simulink model "RI_PMDC_PI"  (R2013b)
settings: Solver=ode45  StartTime=0.0  StopTime=10.0  RelTol=1e-3
libraries: RI_MK x3, simulink x1
settings Model: Creator=Szalay  LastModifiedBy=Szalay

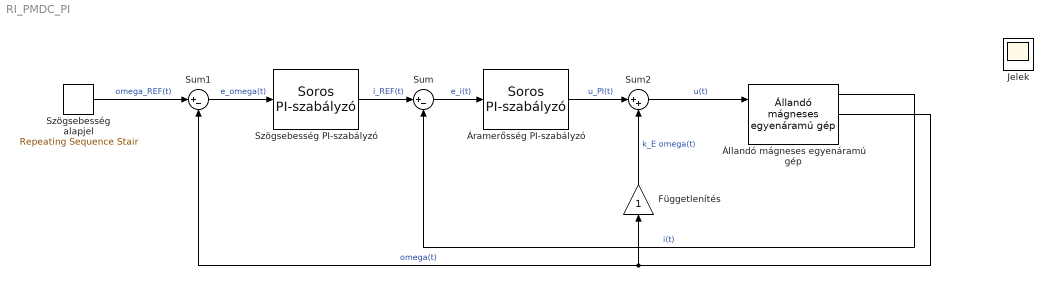
== system RI_PMDC_PI ==
  Függetlenítés : Gain
  Jelek : Scope
  Sum : Sum  Inputs=|+-
  Sum1 : Sum  Inputs=|+-
  Sum2 : Sum  Inputs=|++
  Szögsebesség PI-szabályzó : RI_MK/Soros PI-szabályzó  K_PI=1  T_I=1
  Szögsebesség alapjel : simulink/Sources/Repeating Sequence Stair  OutValues=[3 1 4 2 1].'  tsamp=-1  OutMin=[]  OutMax=[]  OutDataTypeStr=double  OutputDataTypeScalingMode=double  OutDataType=fixdt(0,8)  ConRadixGroup=Best Precision: Vector-wise  OutScaling=2^-12
  Állandó mágneses egyenáramú gép : RI_MK/Állandó mágneses egyenáramú gép  R=1.76  L=658e-6  k_T=68.3e-3  k_E=68.3e-3  J=99.5e-7  B=5.7301e-06  i_0=0  omega_0=0  theta_0=0
  Áramerősség PI-szabályzó : RI_MK/Soros PI-szabályzó  K_PI=1  T_I=1
  wires:
  Sum1/1 -> Szögsebesség PI-szabályzó/1  "e_omega(t)"
  Szögsebesség PI-szabályzó/1 -> Sum/1  "i_REF(t)"
  Sum/1 -> Áramerősség PI-szabályzó/1  "e_i(t)"
  Áramerősség PI-szabályzó/1 -> Sum2/1  "u_PI(t)"
  Sum2/1 -> Állandó mágneses egyenáramú gép/1  "u(t)"
  Állandó mágneses egyenáramú gép/1 -> Sum/2  "i(t)"
  Állandó mágneses egyenáramú gép/2 -> Függetlenítés/1, Sum1/2  "omega(t)"
  Függetlenítés/1 -> Sum2/2  "k_E omega(t)"
  Szögsebesség alapjel/1 -> Sum1/1  "omega_REF(t)"
